simulink model "enclavar"  (R2017a)
settings: Solver=VariableStepAuto  StartTime=0.0  StopTime=10.0  RelTol=1e-3
settings Model: Creator=laure  LastModifiedBy=laure

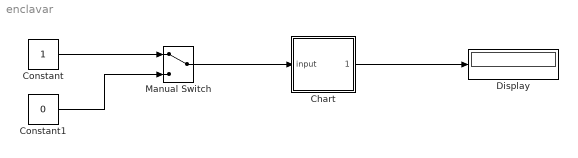
== system enclavar ==
  Chart : Stateflow chart  TreatAsAtomicUnit=on
  Constant : Constant
  Constant1 : Constant  Value=0
  Display : Display
  Manual Switch : ManualSwitch
  wires:
  Manual Switch/1 -> Chart/1(input)
  Chart/1(output) -> Display/1
  Constant/1 -> Manual Switch/1
  Constant1/1 -> Manual Switch/2

== stateflow chart enclavar/Chart ==
  state Up
    during:
    output = 1
  state Down
    during:
    output = 0
  (default) -> Up
  Up -> Down : [input == 1 && after(1, sec)]
  Down -> Up : [input == 1 && after(1, sec)]
  data: output output; input input
